simulink model "ContinuousAndDiscrete"  (R2013b)
settings: Solver=ode45  StartTime=0.0  StopTime=10.0  RelTol=1e-3
libraries: simulink x4
settings Model: Creator=gyurse  LastModifiedBy=gyurse

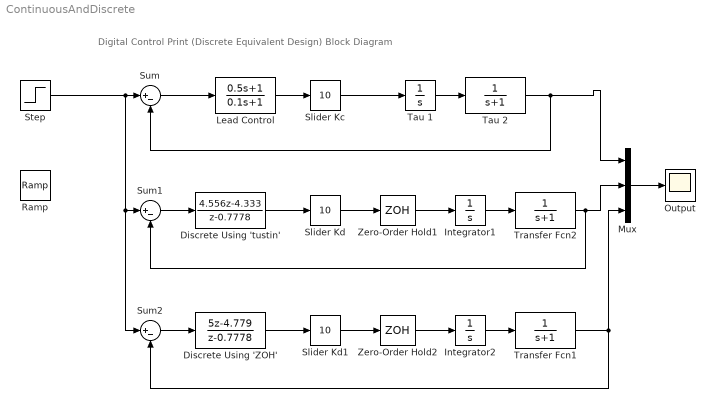
== system ContinuousAndDiscrete ==
  note: Digital Control Print (Discrete Equivalent Design) Block Diagram
  Discrete Using 'ZOH' : DiscreteTransferFcn  Numerator=[5 -4.779]  Denominator=[1 -0.7778]  SampleTime=0.025
  Discrete Using 'tustin' : DiscreteTransferFcn  Numerator=[4.556 -4.333]  Denominator=[1 -0.7778]  SampleTime=0.025
  Integrator1 : Integrator
  Integrator2 : Integrator
  Lead Control : TransferFcn  Numerator=[0.5 1]  Denominator=[0.1 1]
  Mux : Mux  Inputs=3
  Output : Scope
      settings: TimeRange=10  YMin=0  YMax=1.4
  Ramp : simulink/Sources/Ramp  slope=1  start=0  X0=0
  Slider Kc : simulink/Math Operations/Slider Gain  low=0  gain=10  high=10
  Slider Kd : simulink/Math Operations/Slider Gain  low=0  gain=10  high=10
  Slider Kd1 : simulink/Math Operations/Slider Gain  low=0  gain=10  high=10
  Step : Step  SampleTime=0
  Sum : Sum  Inputs=|+-
  Sum1 : Sum  Inputs=|+-
  Sum2 : Sum  Inputs=|+-
  Tau 1 : Integrator
  Tau 2 : TransferFcn  Denominator=[1 1]
  Transfer Fcn1 : TransferFcn  Denominator=[1 1]
  Transfer Fcn2 : TransferFcn  Denominator=[1 1]
  Zero-Order Hold1 : ZeroOrderHold  SampleTime=-1
  Zero-Order Hold2 : ZeroOrderHold  SampleTime=-1
  wires:
  Tau 1/1 -> Tau 2/1
  Integrator1/1 -> Transfer Fcn2/1
  Lead Control/1 -> Slider Kc/1
  Sum/1 -> Lead Control/1
  Step/1 -> Sum2/1, Sum1/1, Sum/1
  Mux/1 -> Output/1
  Tau 2/1 -> Mux/1, Sum/2
  Transfer Fcn2/1 -> Mux/2, Sum1/2
  Sum1/1 -> Discrete Using 'tustin'/1
  Discrete Using 'tustin'/1 -> Slider Kd/1
  Integrator2/1 -> Transfer Fcn1/1
  Transfer Fcn1/1 -> Mux/3, Sum2/2
  Sum2/1 -> Discrete Using 'ZOH'/1
  Discrete Using 'ZOH'/1 -> Slider Kd1/1
  Slider Kd/1 -> Zero-Order Hold1/1
  Zero-Order Hold1/1 -> Integrator1/1
  Slider Kd1/1 -> Zero-Order Hold2/1
  Zero-Order Hold2/1 -> Integrator2/1
  Slider Kc/1 -> Tau 1/1
